simulink model "cruiseSym"  (Simulink 9.3)
settings: Solver=VariableStepAuto  StartTime=0.0  StopTime=100  RelTol=1e-3
values from neighbouring files (symbols this model uses):
  A = 2.4    [constants2.m]
  a3 = 16    [constants2.m]
  B = 0.4    [constants2.m]
  Cd = 0.32    [constants2.m]
  Cr = 0.01    [constants2.m]
  g = 9.8    [constants2.m]
  m = 800    [constants2.m]
  p = 1.3    [constants2.m]
  theta = 0    [constants2.m]
  Tm = 190    [constants2.m]
  wm = 420    [constants2.m]
settings Model: Creator=lucandh1  LastModifiedBy=lucandh1
settings DataIOCC: SaveFormat=Dataset  SignalLoggingSaveFormat=Dataset  ReturnWorkspaceOutputs=on
settings OptimizationCC: LifeSpan=auto
settings DebuggingCC: UnderspecifiedInitializationDetection=Simplified  MergeDetectMultiDrivingBlocksExec=error  FcnCallInpInsideContextMsg=error  SFUnexpectedBacktrackingDiag=error  SFNoUnconditionalDefaultTransitionDiag=error  SFExecutionAtInitializationDiag=warning  ArithmeticOperatorsInVariantConditions=error
settings HardwareCC: ProdBitPerPointer=64  ProdBitPerSizeT=64  ProdBitPerPtrDiffT=64  ProdLargestAtomicFloat=Float  ProdIntDivRoundTo=Zero  ProdEndianess=LittleEndian  ProdWordSize=64  ProdHWDeviceType=Intel->x86-64 (Windows64)
settings ModelReferenceCC: PropagateSignalLabelsOutOfModel=on
settings SFSimCC: SimUseLocalCustomCode=on
settings RTWCC: RTWUseLocalCustomCode=on
settings CodeAppCC: StateflowObjectComments=off
settings GRTTargetCC: TargetLangStandard=C99 (ISO)  CombineOutputUpdateFcns=on  GRTInterface=off
settings ConfigComp: CovMetricSettings=dwe  CovHtmlReporting=off  CovSaveCumulativeToWorkspaceVar=off  CovSaveSingleToWorkspaceVar=off  CovExternalEMLEnable=on

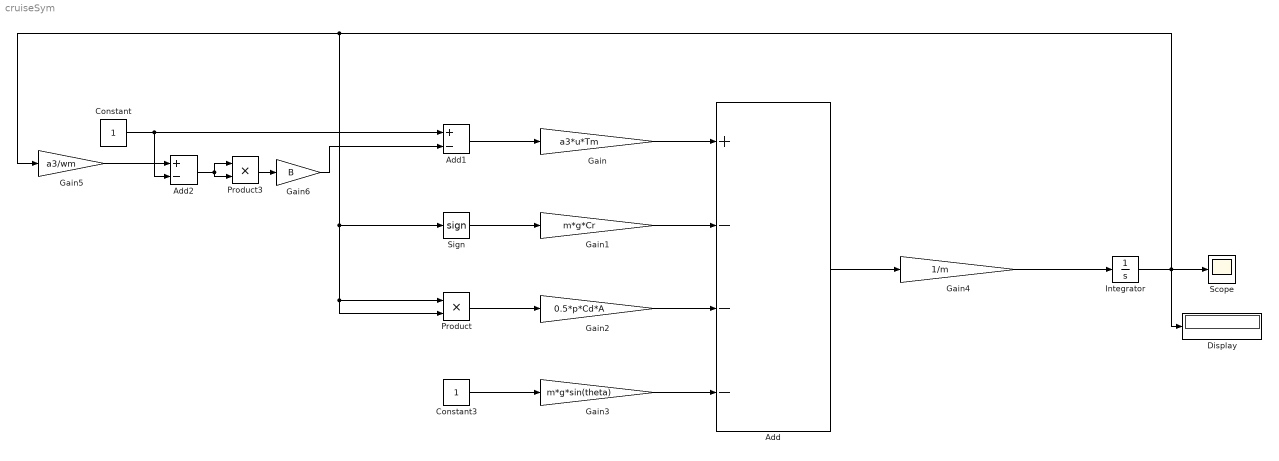
== system cruiseSym ==
  Add : Sum  Inputs=+---
  Add1 : Sum  Inputs=+-
  Add2 : Sum  Inputs=+-
  Constant : Constant
  Constant3 : Constant
  Display : Display
  Gain : Gain  Gain=a3*u*Tm
  Gain1 : Gain  Gain=m*g*Cr
  Gain2 : Gain  Gain=0.5*p*Cd*A
  Gain3 : Gain  Gain=m*g*sin(theta)
  Gain4 : Gain  Gain=1/m
  Gain5 : Gain  Gain=a3/wm
  Gain6 : Gain  Gain=B
  Integrator : Integrator
  Product : Product
  Product3 : Product
  Scope : Scope
  Sign : Signum
  wires:
  Gain3/1 -> Add/4
  Gain2/1 -> Add/3
  Gain1/1 -> Add/2
  Gain/1 -> Add/1
  Add/1 -> Gain4/1
  Gain4/1 -> Integrator/1
  Integrator/1 -> Display/1, Scope/1, Sign/1, Product/1, Product/2, Gain5/1
  Sign/1 -> Gain1/1
  Product/1 -> Gain2/1
  Add1/1 -> Gain/1
  Constant/1 -> Add2/2, Add1/1
  Add2/1 -> Product3/1, Product3/2
  Constant3/1 -> Gain3/1
  Product3/1 -> Gain6/1
  Gain6/1 -> Add1/2
  Gain5/1 -> Add2/1
